simulink model "LQRsim"  (R2018a)
settings: Solver=VariableStepAuto  StartTime=0.0  StopTime=10  RelTol=1e-3
values from neighbouring files (symbols this model uses):
  A = [0 1 0; 0 -b/J_t K/J_t; 0 -K/L -R/L]    [LQRprojekt.m]
  B = [0 ; 0 ; 1/L]    [LQRprojekt.m]
  C = [1 0 0]    [LQRprojekt.m]
  K = lqr(A,B,Q,R)    [LQRprojekt.m]
  L = place(A',C',P)'    [LQRprojekt.m]
  Nbar = rscale(sys_ss,K)    [LQRprojekt.m]
settings Model: Creator=M  LastModifiedBy=M

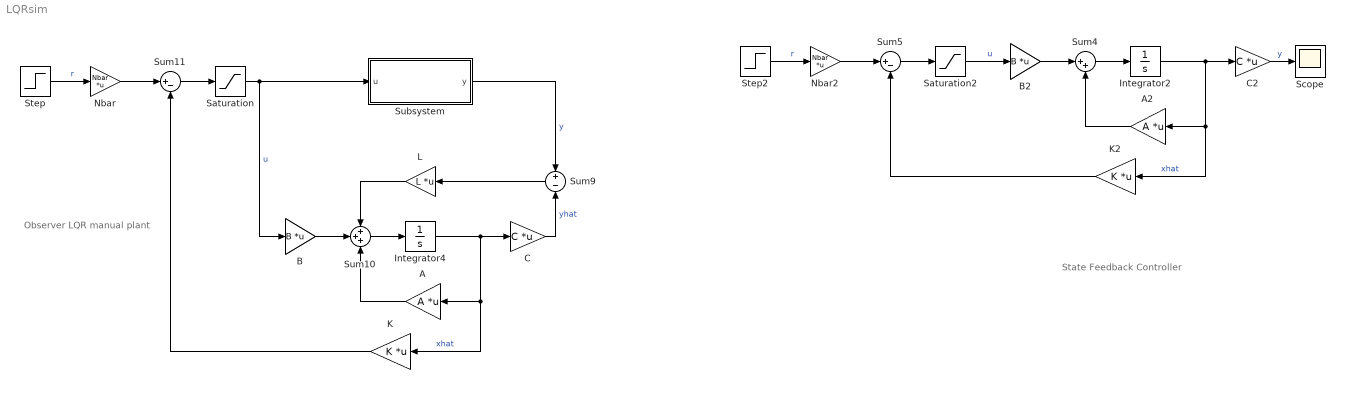
== system LQRsim ==
  note: State Feedback Controller
  note: Observer LQR manual plant
  A : Gain  Gain=A  Multiplication=Matrix(K*u)
  A2 : Gain  Gain=A  Multiplication=Matrix(K*u)
  B : Gain  Gain=B  Multiplication=Matrix(K*u)
  B2 : Gain  Gain=B  Multiplication=Matrix(K*u)
  C : Gain  Gain=C  Multiplication=Matrix(K*u)
  C2 : Gain  Gain=C  Multiplication=Matrix(K*u)
  Integrator2 : Integrator
  Integrator4 : Integrator
  K : Gain  Gain=K  Multiplication=Matrix(K*u)
  K2 : Gain  Gain=K  Multiplication=Matrix(K*u)
  L : Gain  Gain=L  Multiplication=Matrix(K*u)
  Nbar : Gain  Gain=Nbar  Multiplication=Matrix(K*u)
  Nbar2 : Gain  Gain=Nbar  Multiplication=Matrix(K*u)
  Saturation : Saturate  UpperLimit=12  LowerLimit=-12
  Saturation2 : Saturate  UpperLimit=12  LowerLimit=-12
  Scope : Scope
  Step : Step  SampleTime=0
  Step2 : Step  SampleTime=0
  Subsystem : Subsystem
  Sum10 : Sum  Inputs=+++
  Sum11 : Sum  Inputs=|+-
  Sum4 : Sum  Inputs=|++
  Sum5 : Sum  Inputs=|+-
  Sum9 : Sum  Inputs=+-
  wires:
  A/1 -> Sum10/3
  B/1 -> Sum10/2
  Sum9/1 -> L/1
  C/1 -> Sum9/2  "yhat"
  K/1 -> Sum11/2
  L/1 -> Sum10/1
  Sum10/1 -> Integrator4/1
  Integrator4/1 -> C/1, K/1, A/1  "xhat"
  Subsystem/1(y) -> Sum9/1  "y"
  Sum11/1 -> Saturation/1
  Saturation/1 -> B/1, Subsystem/1(u)  "u"
  Nbar/1 -> Sum11/1
  Step/1 -> Nbar/1  "r"
  Sum5/1 -> Saturation2/1
  Saturation2/1 -> B2/1  "u"
  K2/1 -> Sum5/2
  Step2/1 -> Nbar2/1  "r"
  Sum4/1 -> Integrator2/1
  Nbar2/1 -> Sum5/1
  Integrator2/1 -> C2/1, K2/1, A2/1  "xhat"
  A2/1 -> Sum4/2
  B2/1 -> Sum4/1
  C2/1 -> Scope/1  "y"

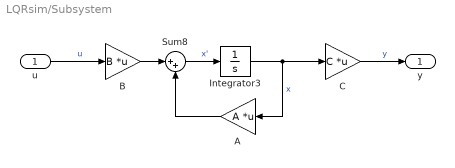
== system LQRsim/Subsystem ==
  u : Inport
  A : Gain  Gain=A  Multiplication=Matrix(K*u)
  B : Gain  Gain=B  Multiplication=Matrix(K*u)
  C : Gain  Gain=C  Multiplication=Matrix(K*u)
  Integrator3 : Integrator
  Sum8 : Sum  Inputs=|++
  y : Outport
  wires:
  u/1 -> B/1  "u"
  Sum8/1 -> Integrator3/1  "x'"
  Integrator3/1 -> A/1, C/1  "x"
  A/1 -> Sum8/2
  B/1 -> Sum8/1
  C/1 -> y/1  "y"
